simulink model "controlSystem_TorqueOptimizer"  (R2021a)
settings: Solver=VariableStepAuto  StartTime=0.0  StopTime=10.0  RelTol=1e-3
undefined symbols (not defined in the file): initialFuel, maxEngineTemp, MaxEngineTorque, maxMotorTemp, maxMotorTorque, MaxMotorTorque, sigbuilder_block
libraries: autolibsharedcoupling x6, autolibpowerinfoutils x4, autolibshared x3, autolibhevctrlrcommon x2, autolibmappedmotor x2, autolibshareddiff x1, autolibtransamt x1, autolibdatasheetbattery x1, autolibsharedmappedengines x1
(part 5 of 5)

== system controlSystem_TorqueOptimizer/Main Controller/Heat Controller ==
  note: Decreases the torque to the motor or engine if they are overheating by the power of the stand-in gain function.
      | This system doesn't make the other motor/engine work harder if one is too hot. Therefore when one is overheated the car instantly loses power, instead of when both are overheated.
  Motor Torque : Inport
  Engine Torque : Inport  Port=2
  Engine Temp Switch : Switch  Criteria=u2 > Threshold  Threshold=maxEngineTemp
  Motor Temp Switch : Switch  Criteria=u2 > Threshold  Threshold=maxMotorTemp
  Signal Builder : Subsystem  Tag=STV Subsys  LoadFcn=sigbuilder_block('load');  StartFcn=sigbuilder_block('start');  StopFcn=sigbuilder_block('stop');  ClipboardFcn=sigbuilder_block('clipboard');  mask(Sigbuilder block){tuvar=[0:10]}
      mask help: Simulink:masks:SigbuilderBlock_MD
      mask init:
      | if ~strcmp(get_param(bdroot(gcbh),'SimulationStatus'),'stopped') tuvar = sigbuilder_block('maskInit'); end
      settings: CopyFcn=sigbuilder_block('copy');  DeleteFcn=sigbuilder_block('delete');  ModelCloseFcn=sigbuilder_block('modelClose');  PreSaveFcn=sigbuilder_block('preSave');  PauseFcn=sigbuilder_block('pause');  ContinueFcn=sigbuilder_block('continue');  NameChangeFcn=sigbuilder_block('namechange');  OpenFcn=sigbuilder_block('open',[411 128.5 543.5 351.5 ]);  CloseFcn=sigbuilder_block('close');
      mask Display: plot(0, 0, 100, 100,[2, 2, 32, 32, 2], [68, 8, 8, 68, 68],[32, 2], [38, 38], [32, 19, 2],[53, 60, 44], [32, 17, 17, 2],[16, 16, 31, 31]);txt = getActiveGroup(gcbh);text(2, 100, txt,'verticalAlignment', 'top');
  place-holder to decrease engine torque : Gain
  place-holder to decrease motor torque : Gain
  Updated Motor Torque : Outport
  Updated Engine Torque : Outport  Port=2
  wires:
  Motor Torque/1 -> place-holder to decrease motor torque/1, Motor Temp Switch/3
  place-holder to decrease motor torque/1 -> Motor Temp Switch/1
  Engine Torque/1 -> place-holder to decrease engine torque/1, Engine Temp Switch/3
  place-holder to decrease engine torque/1 -> Engine Temp Switch/1
  Signal Builder/1(Motor temp) -> Motor Temp Switch/2
  Signal Builder/2(Engine temp) -> Engine Temp Switch/2
  Motor Temp Switch/1 -> Updated Motor Torque/1
  Engine Temp Switch/1 -> Updated Engine Torque/1

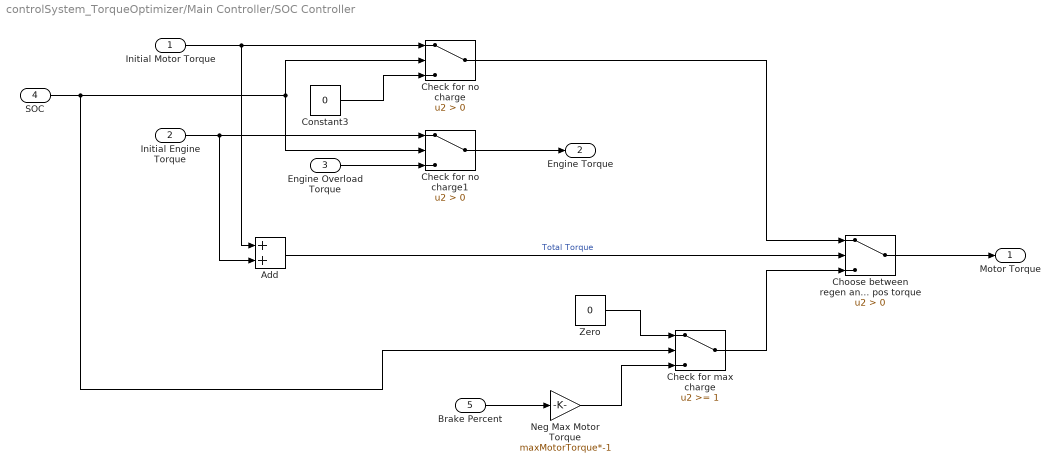
== system controlSystem_TorqueOptimizer/Main Controller/SOC Controller ==
  Initial Motor Torque : Inport
  Initial Engine Torque : Inport  Port=2
  Engine Overload Torque : Inport  Port=3
  SOC : Inport  Port=4
  Brake Percent : Inport  Port=5
  Add : Sum
  Check for max charge : Switch  Threshold=1
  Check for no charge : Switch  Criteria=u2 > Threshold
  Check for no charge1 : Switch  Criteria=u2 > Threshold
  Choose between regen and pos torque : Switch  Criteria=u2 > Threshold
  Constant3 : Constant  Value=0
  Neg Max Motor Torque : Gain  Gain=maxMotorTorque*-1
  Zero : Constant  Value=0  OutDataTypeStr=Inherit: Inherit via back propagation
  Motor Torque : Outport
  Engine Torque : Outport  Port=2
  wires:
  Check for no charge1/1 -> Engine Torque/1
  Engine Overload Torque/1 -> Check for no charge1/3
  Constant3/1 -> Check for no charge/3
  Check for no charge/1 -> Choose between regen and pos torque/1
  Initial Motor Torque/1 -> Add/1, Check for no charge/1
  Initial Engine Torque/1 -> Add/2, Check for no charge1/1
  Brake Percent/1 -> Neg Max Motor Torque/1
  Add/1 -> Choose between regen and pos torque/2  "Total Torque"
  Choose between regen and pos torque/1 -> Motor Torque/1
  SOC/1 -> Check for no charge1/2, Check for no charge/2, Check for max charge/2
  Zero/1 -> Check for max charge/1
  Neg Max Motor Torque/1 -> Check for max charge/3
  Check for max charge/1 -> Choose between regen and pos torque/3

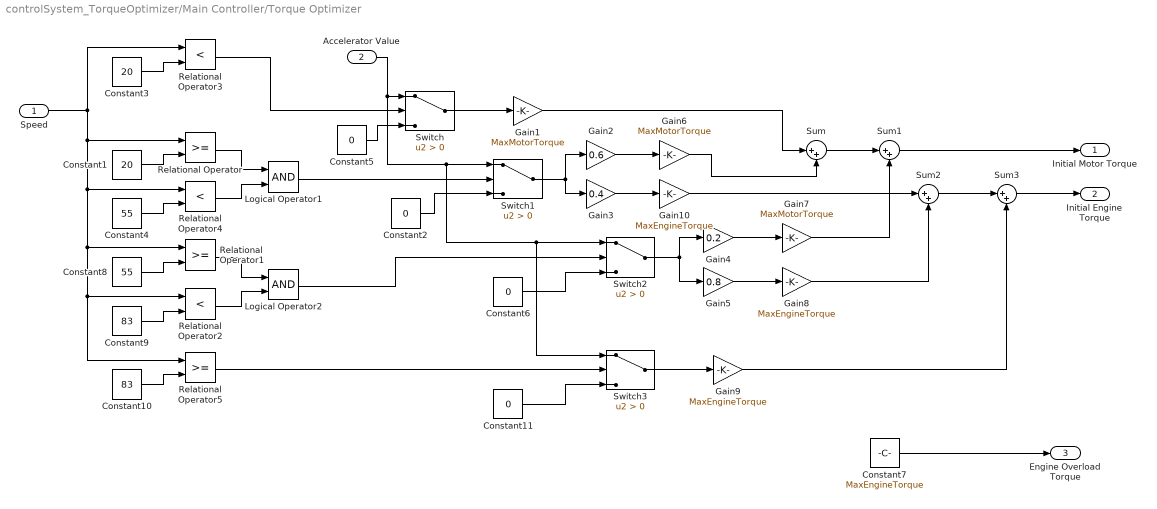
== system controlSystem_TorqueOptimizer/Main Controller/Torque Optimizer ==
  Speed : Inport
  Accelerator Value : Inport  Port=2
  Constant1 : Constant  Value=20
  Constant10 : Constant  Value=83
  Constant{2,5..6,11} (4 alike) : Constant  Value=0
  Constant3 : Constant  Value=20
  Constant4 : Constant  Value=55
  Constant7 : Constant  Value=MaxEngineTorque
  Constant8 : Constant  Value=55
  Constant9 : Constant  Value=83
  Gain1 : Gain  Gain=MaxMotorTorque
  Gain10 : Gain  Gain=MaxEngineTorque
  Gain2 : Gain  Gain=0.6
  Gain3 : Gain  Gain=0.4
  Gain4 : Gain  Gain=0.2
  Gain5 : Gain  Gain=0.8
  Gain6 : Gain  Gain=MaxMotorTorque
  Gain7 : Gain  Gain=MaxMotorTorque
  Gain8 : Gain  Gain=MaxEngineTorque
  Gain9 : Gain  Gain=MaxEngineTorque
  Logical Operator1 : Logic  AllPortsSameDT=off  OutDataTypeStr=boolean
  Logical Operator2 : Logic  AllPortsSameDT=off  OutDataTypeStr=boolean
  Relational Operator : RelationalOperator  OutDataTypeStr=boolean  RndMeth=Simplest
  Relational Operator1 : RelationalOperator  OutDataTypeStr=boolean  RndMeth=Simplest
  Relational Operator2 : RelationalOperator  Operator=<  OutDataTypeStr=boolean  RndMeth=Simplest
  Relational Operator3 : RelationalOperator  Operator=<  OutDataTypeStr=boolean  RndMeth=Simplest
  Relational Operator4 : RelationalOperator  Operator=<  OutDataTypeStr=boolean  RndMeth=Simplest
  Relational Operator5 : RelationalOperator  OutDataTypeStr=boolean  RndMeth=Simplest
  Sum{,1..3} (4 alike) : Sum  Inputs=|++
  Switch{,1..3} (4 alike) : Switch  Criteria=u2 > Threshold
  Initial Motor Torque : Outport
  Initial Engine Torque : Outport  Port=2
  Engine Overload Torque : Outport  Port=3
  wires:
  Constant1/1 -> Relational Operator/2
  Constant3/1 -> Relational Operator3/2
  Constant4/1 -> Relational Operator4/2
  Relational Operator/1 -> Logical Operator1/1
  Relational Operator4/1 -> Logical Operator1/2
  Logical Operator2/1 -> Switch2/2
  Logical Operator1/1 -> Switch1/2
  Relational Operator3/1 -> Switch/2
  Sum/1 -> Sum1/1
  Constant5/1 -> Switch/3
  Constant2/1 -> Switch1/3
  Constant6/1 -> Switch2/3
  Switch2/1 -> Gain5/1, Gain4/1
  Switch1/1 -> Gain3/1, Gain2/1
  Switch/1 -> Gain1/1
  Gain1/1 -> Sum/1
  Gain2/1 -> Gain6/1
  Gain4/1 -> Gain7/1
  Sum1/1 -> Initial Motor Torque/1
  Gain3/1 -> Gain10/1
  Gain5/1 -> Gain8/1
  Constant7/1 -> Engine Overload Torque/1
  Gain6/1 -> Sum/2
  Gain10/1 -> Sum2/1
  Gain7/1 -> Sum1/2
  Gain8/1 -> Sum2/2
  Relational Operator1/1 -> Logical Operator2/1
  Relational Operator2/1 -> Logical Operator2/2
  Constant8/1 -> Relational Operator1/2
  Constant9/1 -> Relational Operator2/2
  Constant10/1 -> Relational Operator5/2
  Speed/1 -> Relational Operator/1, Relational Operator5/1, Relational Operator2/1, Relational Operator1/1, Relational Operator4/1, Relational Operator3/1
  Relational Operator5/1 -> Switch3/2
  Accelerator Value/1 -> Switch3/1, Switch2/1, Switch1/1, Switch/1
  Constant11/1 -> Switch3/3
  Switch3/1 -> Gain9/1
  Gain9/1 -> Sum3/2
  Sum2/1 -> Sum3/1
  Sum3/1 -> Initial Engine Torque/1

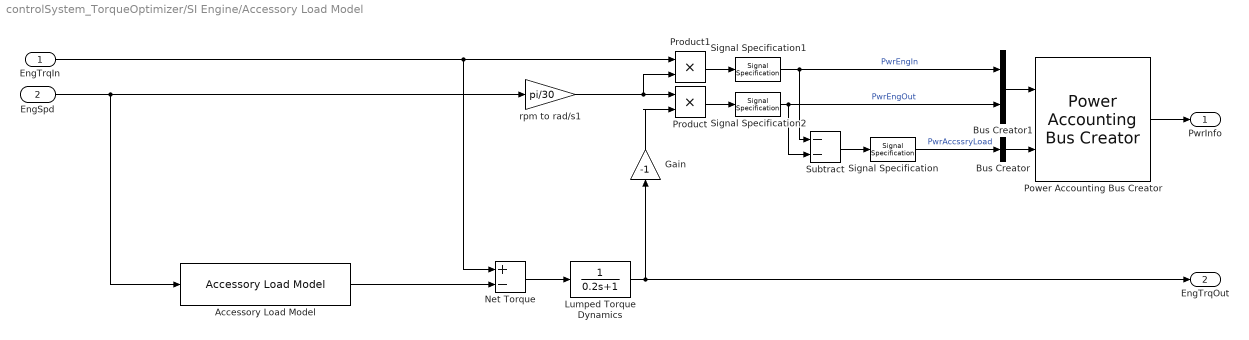
== system controlSystem_TorqueOptimizer/SI Engine/Accessory Load Model ==
  EngTrqIn : Inport
  EngSpd : Inport  Port=2
  Accessory Load Model : autolibhevctrlrcommon/Accessory Load Model  AccPwrTbl=[0 0]  AccSpdBpts=[300 750]
      settings: SourceProductBaseCode=PW
  Bus Creator : BusCreator  Inputs=1
  Bus Creator1 : BusCreator  Inputs=2
  Gain : Gain  Gain=-1
  Lumped Torque Dynamics : TransferFcn  Denominator=[0.2 1]
  Net Torque : Sum  Inputs=+-
  Power Accounting Bus Creator : autolibpowerinfoutils/Power Accounting Bus Creator  AssctBlkSelPopup=Parent  RefBlkName='libraryname/blkname'  PwrTrnsfrdCheckBox=on  PwrNotTrnsfrdCheckBox=on  PwrStoredCheckBox=off  aMode=aMode
      settings: SourceProductBaseCode=PW,DR,MT,UV,VE
  Product : Product
  Product1 : Product
  Signal Specification : SignalSpecification  Unit=W
  Signal Specification1 : SignalSpecification  Unit=W
  Signal Specification2 : SignalSpecification  Unit=W
  Subtract : Sum  Inputs=--
  rpm to rad/s1 : Gain  Gain=pi/30
  PwrInfo : Outport  VectorParamsAs1DForOutWhenUnconnected=off
  EngTrqOut : Outport  Port=2  Unit=N*m  VectorParamsAs1DForOutWhenUnconnected=off
  wires:
  EngSpd/1 -> Accessory Load Model/1, rpm to rad/s1/1
  Lumped Torque Dynamics/1 -> EngTrqOut/1, Gain/1
  Net Torque/1 -> Lumped Torque Dynamics/1
  Bus Creator/1 -> Power Accounting Bus Creator/2
  Bus Creator1/1 -> Power Accounting Bus Creator/1
  EngTrqIn/1 -> Product1/1, Net Torque/1
  Subtract/1 -> Signal Specification/1
  Signal Specification/1 -> Bus Creator/1  "PwrAccssryLoad"
  Power Accounting Bus Creator/1 -> PwrInfo/1
  Product/1 -> Signal Specification2/1
  Product1/1 -> Signal Specification1/1
  rpm to rad/s1/1 -> Product1/2, Product/1
  Signal Specification1/1 -> Subtract/1, Bus Creator1/1  "PwrEngIn"
  Signal Specification2/1 -> Subtract/2, Bus Creator1/2  "PwrEngOut"
  Gain/1 -> Product/2
  Accessory Load Model/1 -> Net Torque/2

== system controlSystem_TorqueOptimizer/Drivetrain/Differential/Rear Axle Compliance 2 ==
  Info : Inport
  Bus Selector : BusSelector  OutputSignals=PwrInfo.PwrTrnsfrd,PwrInfo.PwrNotTrnsfrd,PwrInfo.PwrStored
  Bus Selector1 : BusSelector  OutputSignals=Trq.R,Trq.C
  Power Accounting Bus Creator : autolibpowerinfoutils/Power Accounting Bus Creator  AssctBlkSelPopup=Parent  RefBlkName='libraryname/blkname'  PwrTrnsfrdCheckBox=on  PwrNotTrnsfrdCheckBox=on  PwrStoredCheckBox=on  aMode=aMode
      settings: SourceProductBaseCode=PW,DR,MT,UV,VE
  Terminator : Terminator
  Terminator1 : Terminator
  Terminator2 : Terminator
  Two-Way Connection1 : TwoWayConnection
  Two-Way Connection4 : TwoWayConnection
  R : PMIOPort  Side=Left
  C : PMIOPort  Port=2  Side=Right
  wires:
  Two-Way Connection4/1 -> Terminator/1
  Info/1 -> Bus Selector1/1, Bus Selector/1
  Two-Way Connection1/1 -> Terminator1/1
  Bus Selector1/1 -> Two-Way Connection4/1  "<R>"
  Bus Selector1/2 -> Two-Way Connection1/1  "<C>"
  Power Accounting Bus Creator/1 -> Terminator2/1
  Bus Selector/1 -> Power Accounting Bus Creator/1  "<PwrTrnsfrd>"
  Bus Selector/2 -> Power Accounting Bus Creator/2  "<PwrNotTrnsfrd>"
  Bus Selector/3 -> Power Accounting Bus Creator/3  "<PwrStored>"
  connections:
  R/RConn1 -- Two-Way Connection4/RConn1
  Two-Way Connection1/RConn1 -- C/RConn1

== system controlSystem_TorqueOptimizer/Drivetrain/Transmission/Accessory Load Model ==
  EngTrqIn : Inport
  EngSpd : Inport  Port=2
  Accessory Load Model : autolibhevctrlrcommon/Accessory Load Model  AccPwrTbl=[0 0]  AccSpdBpts=[300 750]
      settings: SourceProductBaseCode=PW
  Lumped Torque Dynamics : TransferFcn  Denominator=[0.2 1]
  Net Torque : Sum  Inputs=+-
  EngTrqOut : Outport  Unit=N*m  VectorParamsAs1DForOutWhenUnconnected=off
  wires:
  EngSpd/1 -> Accessory Load Model/1
  Lumped Torque Dynamics/1 -> EngTrqOut/1
  Net Torque/1 -> Lumped Torque Dynamics/1
  EngTrqIn/1 -> Net Torque/1
  Accessory Load Model/1 -> Net Torque/2

== system controlSystem_TorqueOptimizer/Drivetrain/Transmission/Subsystem ==
  EngSpd : Inport
  AccCmd : Inport  Port=2
  VehSpdFdbk : Inport  Port=3
  Constant : Constant
  Terminator : Terminator
  Terminator1 : Terminator
  Terminator2 : Terminator
  GearCmd : Outport
  wires:
  EngSpd/1 -> Terminator/1
  VehSpdFdbk/1 -> Terminator2/1
  AccCmd/1 -> Terminator1/1
  Constant/1 -> GearCmd/1

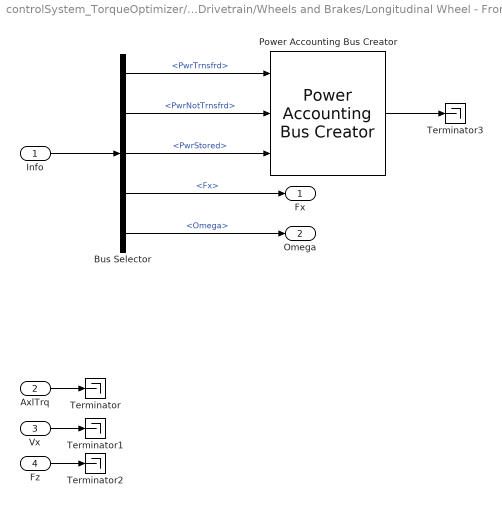
== system controlSystem_TorqueOptimizer/Drivetrain/Wheels and Brakes/Longitudinal Wheel - Front 2 ==
  Info : Inport
  AxlTrq : Inport  Port=2
  Vx : Inport  Port=3
  Fz : Inport  Port=4
  Bus Selector : BusSelector  OutputSignals=PwrInfo.PwrTrnsfrd,PwrInfo.PwrNotTrnsfrd,PwrInfo.PwrStored,Fx,Omega
  Power Accounting Bus Creator : autolibpowerinfoutils/Power Accounting Bus Creator  AssctBlkSelPopup=Parent  RefBlkName='libraryname/blkname'  PwrTrnsfrdCheckBox=on  PwrNotTrnsfrdCheckBox=on  PwrStoredCheckBox=on  aMode=aMode
      settings: SourceProductBaseCode=PW,DR,MT,UV,VE
  Terminator{,1..3} (4 alike) : Terminator
  Fx : Outport  VectorParamsAs1DForOutWhenUnconnected=off
  Omega : Outport  Port=2  VectorParamsAs1DForOutWhenUnconnected=off
  wires:
  AxlTrq/1 -> Terminator/1
  Vx/1 -> Terminator1/1
  Fz/1 -> Terminator2/1
  Info/1 -> Bus Selector/1
  Bus Selector/1 -> Power Accounting Bus Creator/1  "<PwrTrnsfrd>"
  Bus Selector/2 -> Power Accounting Bus Creator/2  "<PwrNotTrnsfrd>"
  Bus Selector/3 -> Power Accounting Bus Creator/3  "<PwrStored>"
  Bus Selector/4 -> Fx/1  "<Fx>"
  Bus Selector/5 -> Omega/1  "<Omega>"
  Power Accounting Bus Creator/1 -> Terminator3/1

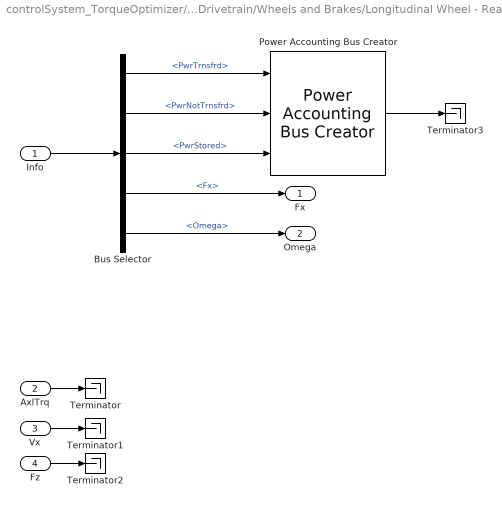
== system controlSystem_TorqueOptimizer/Drivetrain/Wheels and Brakes/Longitudinal Wheel - Rear 2 ==
  Info : Inport
  AxlTrq : Inport  Port=2
  Vx : Inport  Port=3
  Fz : Inport  Port=4
  Bus Selector : BusSelector  OutputSignals=PwrInfo.PwrTrnsfrd,PwrInfo.PwrNotTrnsfrd,PwrInfo.PwrStored,Fx,Omega
  Power Accounting Bus Creator : autolibpowerinfoutils/Power Accounting Bus Creator  AssctBlkSelPopup=Parent  RefBlkName='libraryname/blkname'  PwrTrnsfrdCheckBox=on  PwrNotTrnsfrdCheckBox=on  PwrStoredCheckBox=on  aMode=aMode
      settings: SourceProductBaseCode=PW,DR,MT,UV,VE
  Terminator{,1..3} (4 alike) : Terminator
  Fx : Outport  VectorParamsAs1DForOutWhenUnconnected=off
  Omega : Outport  Port=2  VectorParamsAs1DForOutWhenUnconnected=off
  wires:
  AxlTrq/1 -> Terminator/1
  Vx/1 -> Terminator1/1
  Fz/1 -> Terminator2/1
  Info/1 -> Bus Selector/1
  Bus Selector/1 -> Power Accounting Bus Creator/1  "<PwrTrnsfrd>"
  Bus Selector/2 -> Power Accounting Bus Creator/2  "<PwrNotTrnsfrd>"
  Bus Selector/3 -> Power Accounting Bus Creator/3  "<PwrStored>"
  Bus Selector/4 -> Fx/1  "<Fx>"
  Bus Selector/5 -> Omega/1  "<Omega>"
  Power Accounting Bus Creator/1 -> Terminator3/1

== system controlSystem_TorqueOptimizer/Main Controller/Heat Controller/Signal Builder ==
  Demux : Demux  Tag=STV Demux  Outputs=2
      settings: DisplayOption=none
  FromWs : FromWorkspace  Tag=STV FromWs  VariableName=tuvar
      SigBuilderData=|
      | common.afterFinalStr = 'Extrapolate'
      | common.sampleTime = 0
      | dataSet.timeRange = [0 10]
      | dataSet.name = 'Temperature Signals'
      | sbobj.Groups.Name = 'Temperature Signals'
      | sbobj.Groups.Signals(1).Name = 'Motor temp'
      | sbobj.Groups.Signals(1).XData = [0 10]
      | sbobj.Groups.Signals(1).YData = [0 0]
      | sbobj.Groups.Signals(2).Name = 'Engine temp'
      | sbobj.Groups.Signals(2).XData = [0 10]
      | sbobj.Groups.Signals(2).YData = [0 0]
  Motor temp : Outport  Tag=STV Outport
  Engine temp : Outport  Tag=STV Outport  Port=2
  wires:
  FromWs/1 -> Demux/1
  Demux/1 -> Motor temp/1
  Demux/2 -> Engine temp/1
